simulink model "System_TC6"  (R2015b)
settings: Solver=FixedStepAuto  StartTime=0.0  StopTime=20  FixedStep=0.1  RelTol=1e-3
model workspace: external: MAT-File System_TC6.mat (data not in the file)
libraries: libTLAsserts x16, libAsserts x10
settings Model: Creator=Deepak  LastModifiedBy=Deepak

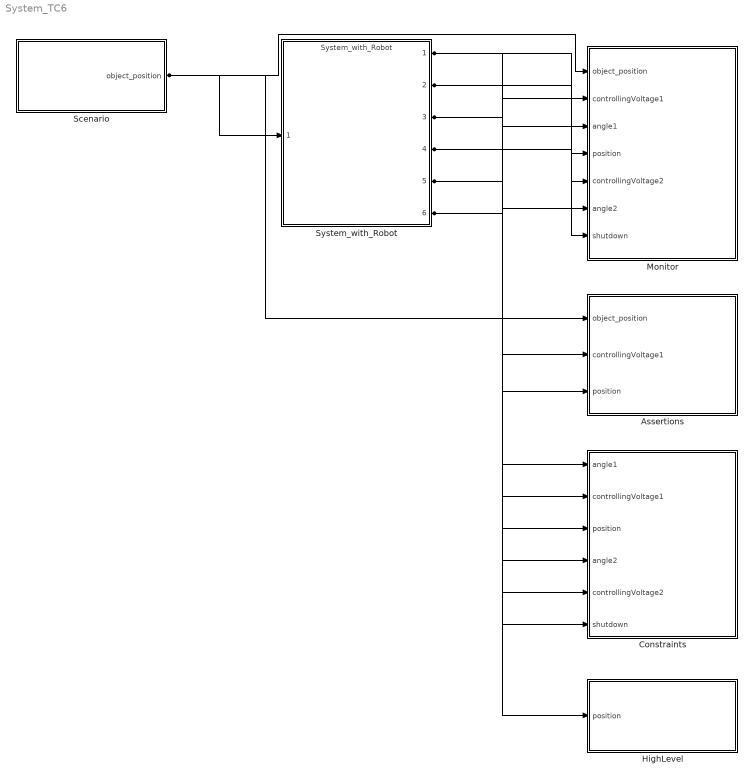
== system System_TC6 ==
  Assertions : Subsystem
  Constraints : Subsystem
  HighLevel : Subsystem
  Monitor : Subsystem
  Scenario : Subsystem
  System_with_Robot : ModelReference  ModelNameDialog=System_with_Robot  SimulationMode=Normal  ModelReferenceVersion=1.26  CopyOfModelName=System_with_Robot
  wires:
  Scenario/1(object_position) -> System_with_Robot/1, Monitor/1(object_position), Assertions/1(object_position)
  System_with_Robot/3 -> Monitor/2(controllingVoltage1), Assertions/2(controllingVoltage1), Constraints/2(controllingVoltage1)
  System_with_Robot/5 -> Monitor/3(angle1), Constraints/1(angle1)
  System_with_Robot/1 -> Monitor/4(position), Assertions/3(position), Constraints/3(position), HighLevel/1(position)
  System_with_Robot/4 -> Monitor/5(controllingVoltage2), Constraints/5(controllingVoltage2)
  System_with_Robot/6 -> Monitor/6(angle2), Constraints/4(angle2)
  System_with_Robot/2 -> Monitor/7(shutdown), Constraints/6(shutdown)

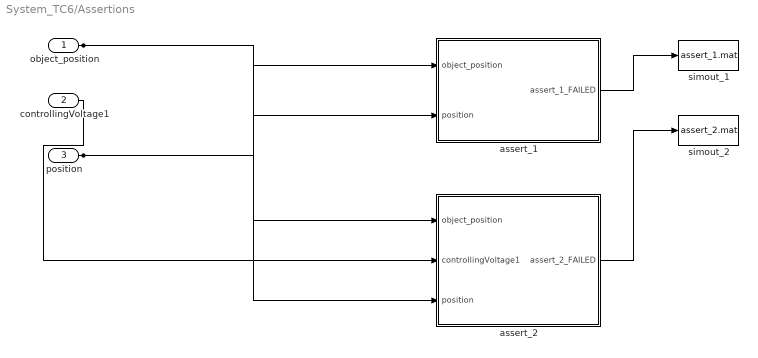
== system System_TC6/Assertions ==
  object_position : Inport
  controllingVoltage1 : Inport  Port=2
  position : Inport  Port=3
  assert_1 : Subsystem
  assert_2 : Subsystem
  simout_1 : ToFile  Filename=assert_1.mat  MatrixName=assert_1  SaveFormat=Timeseries
  simout_2 : ToFile  Filename=assert_2.mat  MatrixName=assert_2  SaveFormat=Timeseries
  wires:
  object_position/1 -> assert_1/1(object_position), assert_2/1(object_position)
  position/1 -> assert_1/2(position), assert_2/3(position)
  assert_1/1(assert_1_FAILED) -> simout_1/1
  controllingVoltage1/1 -> assert_2/2(controllingVoltage1)
  assert_2/1(assert_2_FAILED) -> simout_2/1

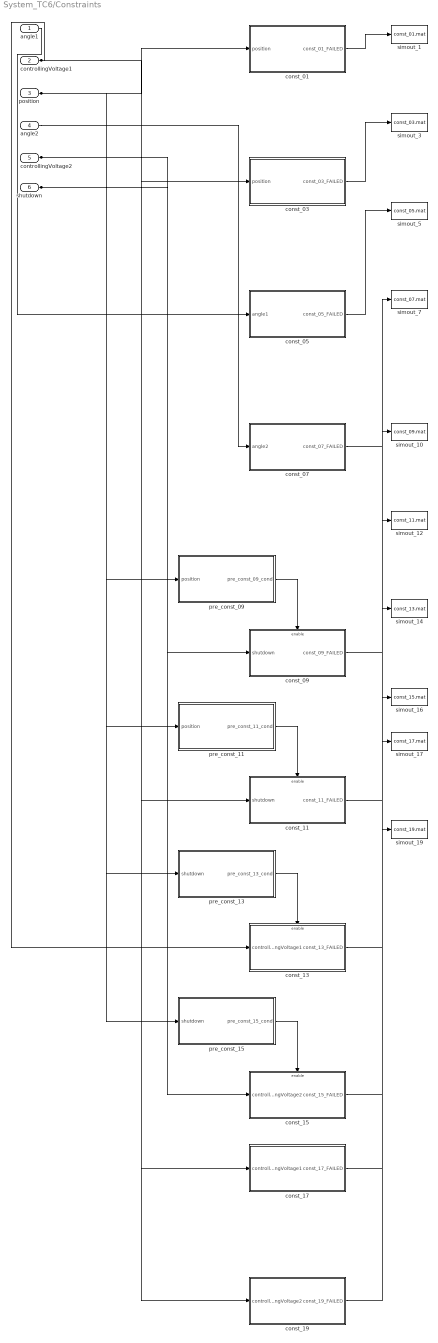
== system System_TC6/Constraints ==
  angle1 : Inport
  controllingVoltage1 : Inport  Port=2
  position : Inport  Port=3
  angle2 : Inport  Port=4
  controllingVoltage2 : Inport  Port=5
  shutdown : Inport  Port=6
  const_01 : Subsystem
  const_03 : Subsystem
  const_05 : Subsystem
  const_07 : Subsystem
  const_09 : Subsystem
  const_11 : Subsystem
  const_13 : Subsystem
  const_15 : Subsystem
  const_17 : Subsystem
  const_19 : Subsystem
  pre_const_09 : Subsystem
  pre_const_11 : Subsystem
  pre_const_13 : Subsystem
  pre_const_15 : Subsystem
  simout_1 : ToFile  Filename=const_01.mat  MatrixName=const_01  SaveFormat=Timeseries
  simout_10 : ToFile  Filename=const_09.mat  MatrixName=const_09  SaveFormat=Timeseries
  simout_12 : ToFile  Filename=const_11.mat  MatrixName=const_11  SaveFormat=Timeseries
  simout_14 : ToFile  Filename=const_13.mat  MatrixName=const_13  SaveFormat=Timeseries
  simout_16 : ToFile  Filename=const_15.mat  MatrixName=const_15  SaveFormat=Timeseries
  simout_17 : ToFile  Filename=const_17.mat  MatrixName=const_17  SaveFormat=Timeseries
  simout_19 : ToFile  Filename=const_19.mat  MatrixName=const_19  SaveFormat=Timeseries
  simout_3 : ToFile  Filename=const_03.mat  MatrixName=const_03  SaveFormat=Timeseries
  simout_5 : ToFile  Filename=const_05.mat  MatrixName=const_05  SaveFormat=Timeseries
  simout_7 : ToFile  Filename=const_07.mat  MatrixName=const_07  SaveFormat=Timeseries
  wires:
  position/1 -> const_01/1(position), const_03/1(position), pre_const_09/1(position), pre_const_11/1(position)
  const_01/1(const_01_FAILED) -> simout_1/1
  const_03/1(const_03_FAILED) -> simout_3/1
  angle1/1 -> const_05/1(angle1)
  const_05/1(const_05_FAILED) -> simout_5/1
  angle2/1 -> const_07/1(angle2)
  const_07/1(const_07_FAILED) -> simout_7/1
  pre_const_09/1(pre_const_09_cond) -> const_09/Enable
  shutdown/1 -> const_09/1(shutdown), const_11/1(shutdown), pre_const_13/1(shutdown), pre_const_15/1(shutdown)
  const_09/1(const_09_FAILED) -> simout_10/1
  pre_const_11/1(pre_const_11_cond) -> const_11/Enable
  const_11/1(const_11_FAILED) -> simout_12/1
  pre_const_13/1(pre_const_13_cond) -> const_13/Enable
  controllingVoltage1/1 -> const_13/1(controllingVoltage1), const_17/1(controllingVoltage1)
  const_13/1(const_13_FAILED) -> simout_14/1
  pre_const_15/1(pre_const_15_cond) -> const_15/Enable
  controllingVoltage2/1 -> const_15/1(controllingVoltage2), const_19/1(controllingVoltage2)
  const_15/1(const_15_FAILED) -> simout_16/1
  const_17/1(const_17_FAILED) -> simout_17/1
  const_19/1(const_19_FAILED) -> simout_19/1

== system System_TC6/HighLevel ==
  position : Inport
  highlevel_1 : Subsystem
  simout_1 : ToFile  Filename=highlevel_1.mat  MatrixName=highlevel_1  SaveFormat=Timeseries
  wires:
  position/1 -> highlevel_1/1(position)
  highlevel_1/1(highlevel_1_FAILED) -> simout_1/1

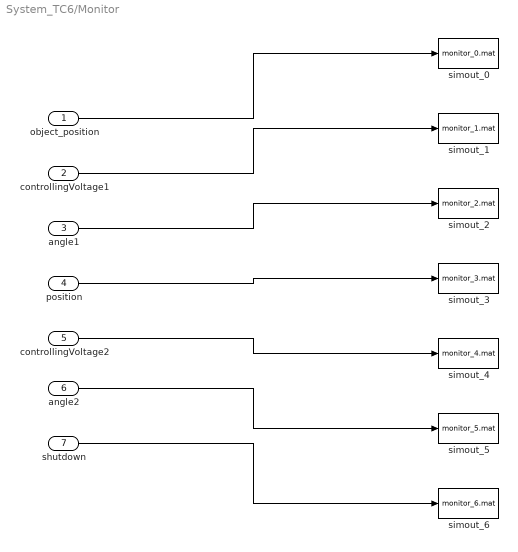
== system System_TC6/Monitor ==
  object_position : Inport
  controllingVoltage1 : Inport  Port=2
  angle1 : Inport  Port=3
  position : Inport  Port=4
  controllingVoltage2 : Inport  Port=5
  angle2 : Inport  Port=6
  shutdown : Inport  Port=7
  simout_0 : ToFile  Filename=monitor_0.mat  MatrixName=object_position  SaveFormat=Timeseries
  simout_1 : ToFile  Filename=monitor_1.mat  MatrixName=controllingVoltage1  SaveFormat=Timeseries
  simout_2 : ToFile  Filename=monitor_2.mat  MatrixName=angle1  SaveFormat=Timeseries
  simout_3 : ToFile  Filename=monitor_3.mat  MatrixName=position  SaveFormat=Timeseries
  simout_4 : ToFile  Filename=monitor_4.mat  MatrixName=controllingVoltage2  SaveFormat=Timeseries
  simout_5 : ToFile  Filename=monitor_5.mat  MatrixName=angle2  SaveFormat=Timeseries
  simout_6 : ToFile  Filename=monitor_6.mat  MatrixName=shutdown  SaveFormat=Timeseries
  wires:
  object_position/1 -> simout_0/1
  controllingVoltage1/1 -> simout_1/1
  angle1/1 -> simout_2/1
  position/1 -> simout_3/1
  controllingVoltage2/1 -> simout_4/1
  angle2/1 -> simout_5/1
  shutdown/1 -> simout_6/1

== system System_TC6/Scenario ==
  Scenario : Stateflow chart  TreatAsAtomicUnit=on
  clock : Clock
  object_position : Outport
  wires:
  Scenario/1(object_position) -> object_position/1
  clock/1 -> Scenario/1(clk)

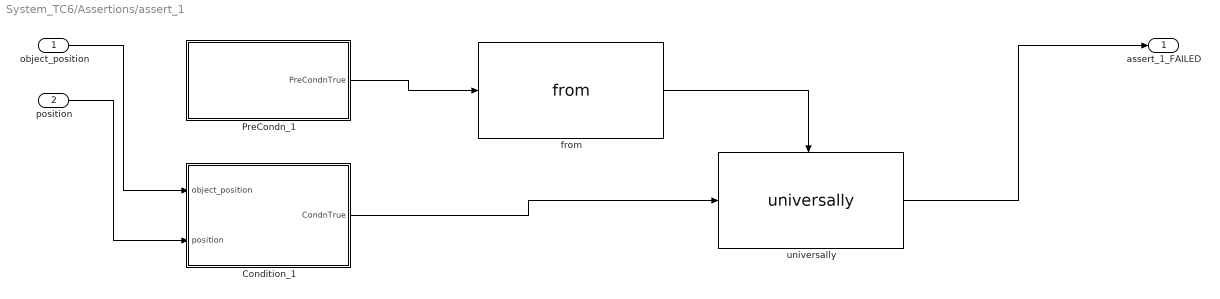
== system System_TC6/Assertions/assert_1 ==
  object_position : Inport
  position : Inport  Port=2
  Condition_1 : Subsystem
  PreCondn_1 : Subsystem
  from : libTLAsserts/from
  universally : libTLAsserts/universally
  assert_1_FAILED : Outport
  wires:
  object_position/1 -> Condition_1/1(object_position)
  position/1 -> Condition_1/2(position)
  PreCondn_1/1(PreCondnTrue) -> from/1
  Condition_1/1(CondnTrue) -> universally/1
  from/1 -> universally/Enable
  universally/1 -> assert_1_FAILED/1

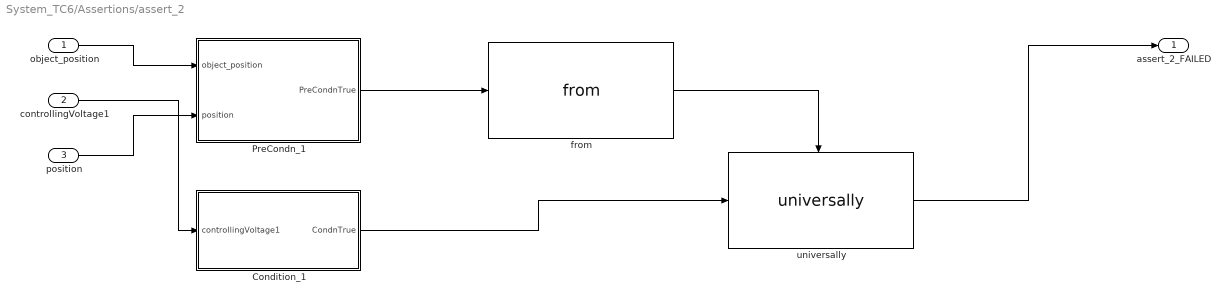
== system System_TC6/Assertions/assert_2 ==
  object_position : Inport
  controllingVoltage1 : Inport  Port=2
  position : Inport  Port=3
  Condition_1 : Subsystem
  PreCondn_1 : Subsystem
  from : libTLAsserts/from
  universally : libTLAsserts/universally
  assert_2_FAILED : Outport
  wires:
  object_position/1 -> PreCondn_1/1(object_position)
  position/1 -> PreCondn_1/2(position)
  controllingVoltage1/1 -> Condition_1/1(controllingVoltage1)
  PreCondn_1/1(PreCondnTrue) -> from/1
  Condition_1/1(CondnTrue) -> universally/1
  from/1 -> universally/Enable
  universally/1 -> assert_2_FAILED/1

== system System_TC6/Constraints/const_01 ==
  position : Inport
  Condition_1 : Subsystem
  globally : libTLAsserts/globally
  universally : libTLAsserts/universally
  const_01_FAILED : Outport
  wires:
  position/1 -> Condition_1/1(position)
  Condition_1/1(CondnTrue) -> universally/1
  globally/1 -> universally/Enable
  universally/1 -> const_01_FAILED/1

== system System_TC6/Constraints/const_03 ==
  position : Inport
  Condition_1 : Subsystem
  globally : libTLAsserts/globally
  universally : libTLAsserts/universally
  const_03_FAILED : Outport
  wires:
  position/1 -> Condition_1/1(position)
  Condition_1/1(CondnTrue) -> universally/1
  globally/1 -> universally/Enable
  universally/1 -> const_03_FAILED/1

== system System_TC6/Constraints/const_05 ==
  angle1 : Inport
  Condition_1 : Subsystem
  globally : libTLAsserts/globally
  universally : libTLAsserts/universally
  const_05_FAILED : Outport
  wires:
  angle1/1 -> Condition_1/1(angle1)
  Condition_1/1(CondnTrue) -> universally/1
  globally/1 -> universally/Enable
  universally/1 -> const_05_FAILED/1

== system System_TC6/Constraints/const_07 ==
  angle2 : Inport
  Condition_1 : Subsystem
  globally : libTLAsserts/globally
  universally : libTLAsserts/universally
  const_07_FAILED : Outport
  wires:
  angle2/1 -> Condition_1/1(angle2)
  Condition_1/1(CondnTrue) -> universally/1
  globally/1 -> universally/Enable
  universally/1 -> const_07_FAILED/1

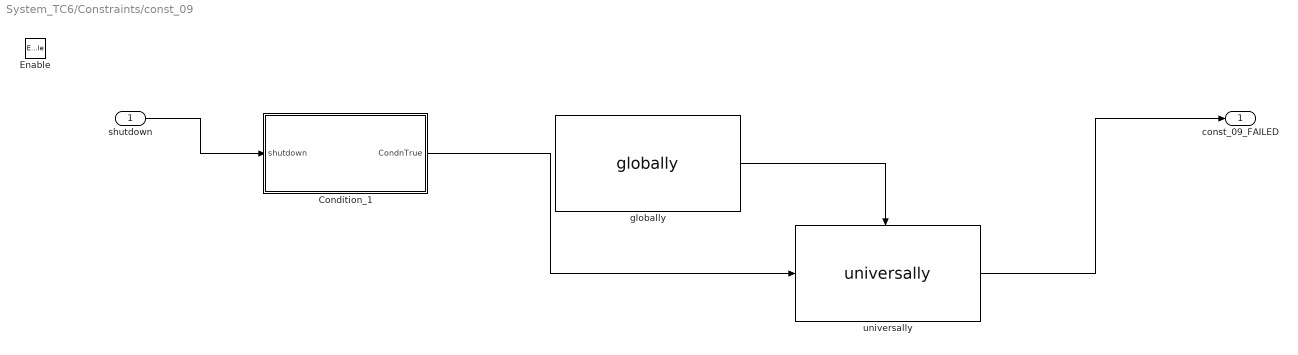
== system System_TC6/Constraints/const_09 ==
  shutdown : Inport
  Enable : EnablePort
  Condition_1 : Subsystem
  globally : libAsserts/globally
  universally : libAsserts/universally
  const_09_FAILED : Outport
  wires:
  shutdown/1 -> Condition_1/1(shutdown)
  Condition_1/1(CondnTrue) -> universally/1
  universally/1 -> const_09_FAILED/1
  globally/1 -> universally/Enable

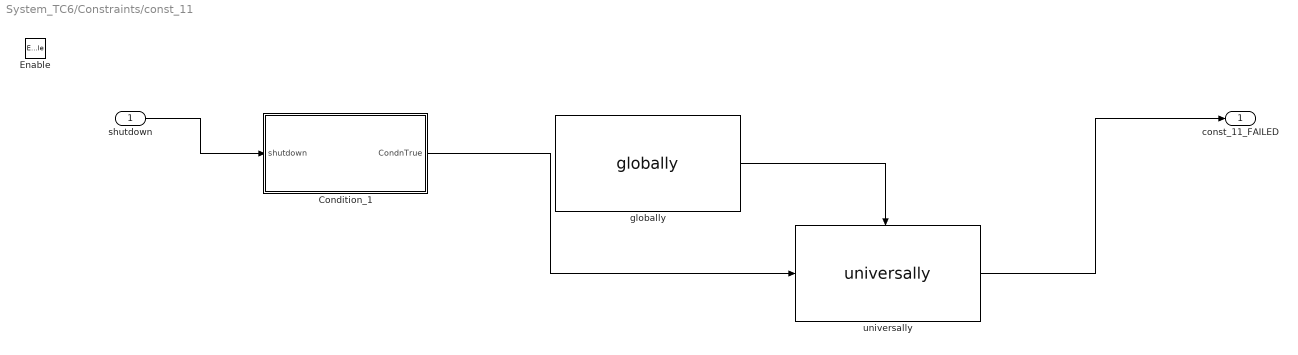
== system System_TC6/Constraints/const_11 ==
  shutdown : Inport
  Enable : EnablePort
  Condition_1 : Subsystem
  globally : libAsserts/globally
  universally : libAsserts/universally
  const_11_FAILED : Outport
  wires:
  shutdown/1 -> Condition_1/1(shutdown)
  Condition_1/1(CondnTrue) -> universally/1
  universally/1 -> const_11_FAILED/1
  globally/1 -> universally/Enable

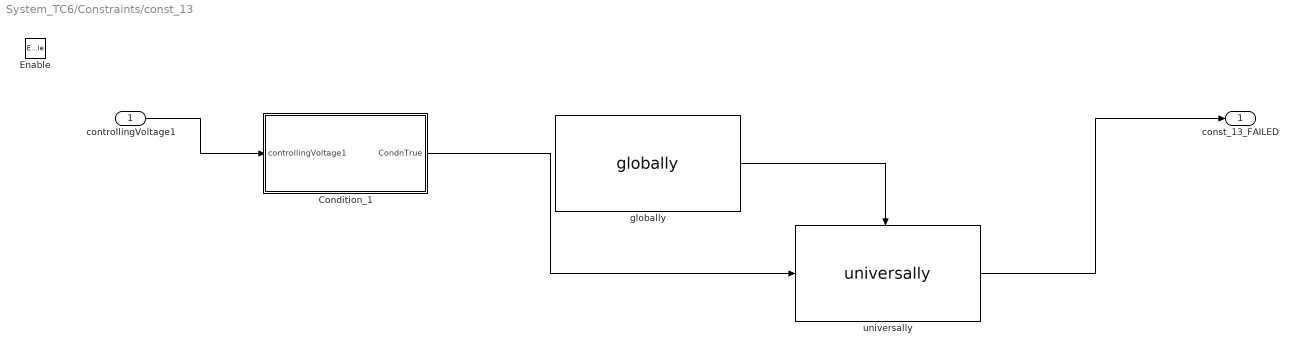
== system System_TC6/Constraints/const_13 ==
  controllingVoltage1 : Inport
  Enable : EnablePort
  Condition_1 : Subsystem
  globally : libAsserts/globally
  universally : libAsserts/universally
  const_13_FAILED : Outport
  wires:
  controllingVoltage1/1 -> Condition_1/1(controllingVoltage1)
  Condition_1/1(CondnTrue) -> universally/1
  universally/1 -> const_13_FAILED/1
  globally/1 -> universally/Enable

== system System_TC6/Constraints/const_15 ==
  controllingVoltage2 : Inport
  Enable : EnablePort
  Condition_1 : Subsystem
  globally : libAsserts/globally
  universally : libAsserts/universally
  const_15_FAILED : Outport
  wires:
  controllingVoltage2/1 -> Condition_1/1(controllingVoltage2)
  Condition_1/1(CondnTrue) -> universally/1
  universally/1 -> const_15_FAILED/1
  globally/1 -> universally/Enable

== system System_TC6/Constraints/const_17 ==
  controllingVoltage1 : Inport
  Condition_1 : Subsystem
  globally : libTLAsserts/globally
  universally : libTLAsserts/universally
  const_17_FAILED : Outport
  wires:
  controllingVoltage1/1 -> Condition_1/1(controllingVoltage1)
  Condition_1/1(CondnTrue) -> universally/1
  globally/1 -> universally/Enable
  universally/1 -> const_17_FAILED/1

== system System_TC6/Constraints/const_19 ==
  controllingVoltage2 : Inport
  Condition_1 : Subsystem
  globally : libTLAsserts/globally
  universally : libTLAsserts/universally
  const_19_FAILED : Outport
  wires:
  controllingVoltage2/1 -> Condition_1/1(controllingVoltage2)
  Condition_1/1(CondnTrue) -> universally/1
  globally/1 -> universally/Enable
  universally/1 -> const_19_FAILED/1

== system System_TC6/Constraints/pre_const_09 ==
  position : Inport
  GreaterExpression_3.0_1.0 : RelationalOperator  Operator=>  OutDataTypeStr=boolean
  NumberLiteral_1.0_1.0 : Constant
  NumberLiteral_1.0_2.0 : Constant  Value=6
  PortItemRefTarget_1.0_1.0 : MultiPortSwitch  Inputs=1
  pre_const_09_cond : Outport
  wires:
  NumberLiteral_1.0_1.0/1 -> PortItemRefTarget_1.0_1.0/1
  position/1 -> PortItemRefTarget_1.0_1.0/2
  PortItemRefTarget_1.0_1.0/1 -> GreaterExpression_3.0_1.0/1
  NumberLiteral_1.0_2.0/1 -> GreaterExpression_3.0_1.0/2
  GreaterExpression_3.0_1.0/1 -> pre_const_09_cond/1

== system System_TC6/Constraints/pre_const_11 ==
  position : Inport
  GreaterExpression_3.0_1.0 : RelationalOperator  Operator=>  OutDataTypeStr=boolean
  NumberLiteral_1.0_1.0 : Constant  Value=2
  NumberLiteral_1.0_2.0 : Constant  Value=6
  PortItemRefTarget_1.0_1.0 : MultiPortSwitch  Inputs=1
  pre_const_11_cond : Outport
  wires:
  NumberLiteral_1.0_1.0/1 -> PortItemRefTarget_1.0_1.0/1
  position/1 -> PortItemRefTarget_1.0_1.0/2
  PortItemRefTarget_1.0_1.0/1 -> GreaterExpression_3.0_1.0/1
  NumberLiteral_1.0_2.0/1 -> GreaterExpression_3.0_1.0/2
  GreaterExpression_3.0_1.0/1 -> pre_const_11_cond/1

== system System_TC6/Constraints/pre_const_13 ==
  shutdown : Inport
  pre_const_13_cond : Outport
  wires:
  shutdown/1 -> pre_const_13_cond/1

== system System_TC6/Constraints/pre_const_15 ==
  shutdown : Inport
  pre_const_15_cond : Outport
  wires:
  shutdown/1 -> pre_const_15_cond/1

== system System_TC6/HighLevel/highlevel_1 ==
  position : Inport
  Condition_1 : Subsystem
  globally : libAsserts/globally
  universally : libAsserts/universally
  highlevel_1_FAILED : Outport
  wires:
  position/1 -> Condition_1/1(position)
  Condition_1/1(CondnTrue) -> universally/1
  universally/1 -> highlevel_1_FAILED/1
  globally/1 -> universally/Enable

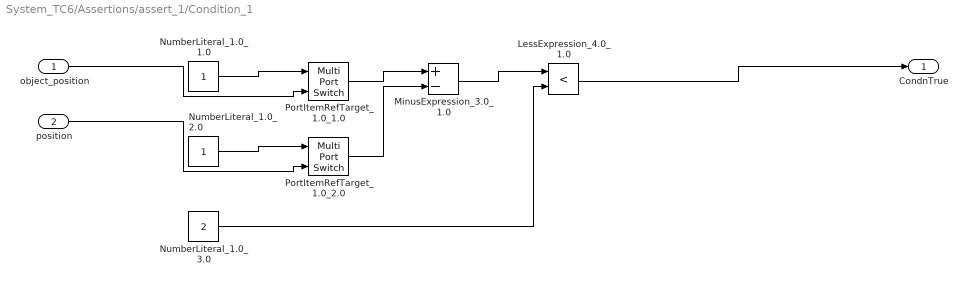
== system System_TC6/Assertions/assert_1/Condition_1 ==
  object_position : Inport
  position : Inport  Port=2
  LessExpression_4.0_1.0 : RelationalOperator  Operator=<  OutDataTypeStr=boolean
  MinusExpression_3.0_1.0 : Sum  Inputs=+-
  NumberLiteral_1.0_1.0 : Constant
  NumberLiteral_1.0_2.0 : Constant
  NumberLiteral_1.0_3.0 : Constant  Value=2
  PortItemRefTarget_1.0_1.0 : MultiPortSwitch  Inputs=1
  PortItemRefTarget_1.0_2.0 : MultiPortSwitch  Inputs=1
  CondnTrue : Outport
  wires:
  NumberLiteral_1.0_1.0/1 -> PortItemRefTarget_1.0_1.0/1
  object_position/1 -> PortItemRefTarget_1.0_1.0/2
  NumberLiteral_1.0_2.0/1 -> PortItemRefTarget_1.0_2.0/1
  position/1 -> PortItemRefTarget_1.0_2.0/2
  PortItemRefTarget_1.0_1.0/1 -> MinusExpression_3.0_1.0/1
  PortItemRefTarget_1.0_2.0/1 -> MinusExpression_3.0_1.0/2
  MinusExpression_3.0_1.0/1 -> LessExpression_4.0_1.0/1
  NumberLiteral_1.0_3.0/1 -> LessExpression_4.0_1.0/2
  LessExpression_4.0_1.0/1 -> CondnTrue/1

== system System_TC6/Assertions/assert_1/PreCondn_1 ==
  AnnotatedExpression_2.0_1.0 : RelationalOperator  OutDataTypeStr=boolean
  NumberLiteral_1.0_1.0 : Constant  Value=5
  clock : Clock
  PreCondnTrue : Outport
  wires:
  clock/1 -> AnnotatedExpression_2.0_1.0/1
  NumberLiteral_1.0_1.0/1 -> AnnotatedExpression_2.0_1.0/2
  AnnotatedExpression_2.0_1.0/1 -> PreCondnTrue/1

== system System_TC6/Assertions/assert_2/Condition_1 ==
  controllingVoltage1 : Inport
  LessExpression_2.0_1.0 : RelationalOperator  Operator=<  OutDataTypeStr=boolean
  NumberLiteral_1.0_1.0 : Constant  Value=2
  CondnTrue : Outport
  wires:
  controllingVoltage1/1 -> LessExpression_2.0_1.0/1
  NumberLiteral_1.0_1.0/1 -> LessExpression_2.0_1.0/2
  LessExpression_2.0_1.0/1 -> CondnTrue/1

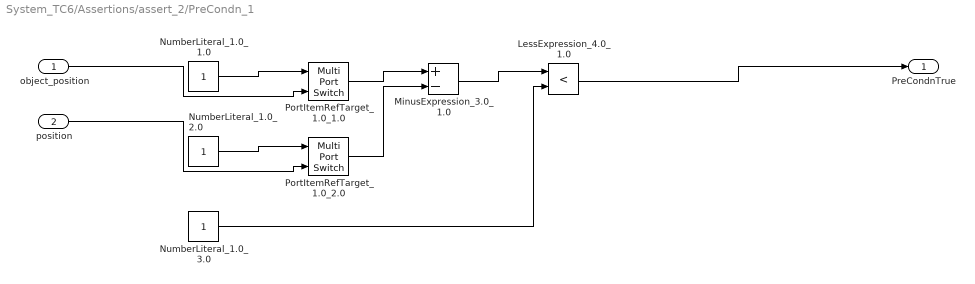
== system System_TC6/Assertions/assert_2/PreCondn_1 ==
  object_position : Inport
  position : Inport  Port=2
  LessExpression_4.0_1.0 : RelationalOperator  Operator=<  OutDataTypeStr=boolean
  MinusExpression_3.0_1.0 : Sum  Inputs=+-
  NumberLiteral_1.0_1.0 : Constant
  NumberLiteral_1.0_2.0 : Constant
  NumberLiteral_1.0_3.0 : Constant
  PortItemRefTarget_1.0_1.0 : MultiPortSwitch  Inputs=1
  PortItemRefTarget_1.0_2.0 : MultiPortSwitch  Inputs=1
  PreCondnTrue : Outport
  wires:
  NumberLiteral_1.0_1.0/1 -> PortItemRefTarget_1.0_1.0/1
  object_position/1 -> PortItemRefTarget_1.0_1.0/2
  NumberLiteral_1.0_2.0/1 -> PortItemRefTarget_1.0_2.0/1
  position/1 -> PortItemRefTarget_1.0_2.0/2
  PortItemRefTarget_1.0_1.0/1 -> MinusExpression_3.0_1.0/1
  PortItemRefTarget_1.0_2.0/1 -> MinusExpression_3.0_1.0/2
  MinusExpression_3.0_1.0/1 -> LessExpression_4.0_1.0/1
  NumberLiteral_1.0_3.0/1 -> LessExpression_4.0_1.0/2
  LessExpression_4.0_1.0/1 -> PreCondnTrue/1

== system System_TC6/Constraints/const_01/Condition_1 ==
  position : Inport
  LessEqualsExpression_3.0_1.0 : RelationalOperator  Operator=<=  OutDataTypeStr=boolean
  NumberLiteral_1.0_1.0 : Constant
  NumberLiteral_1.0_2.0 : Constant  Value=6
  PortItemRefTarget_1.0_1.0 : MultiPortSwitch  Inputs=1
  CondnTrue : Outport
  wires:
  NumberLiteral_1.0_1.0/1 -> PortItemRefTarget_1.0_1.0/1
  position/1 -> PortItemRefTarget_1.0_1.0/2
  PortItemRefTarget_1.0_1.0/1 -> LessEqualsExpression_3.0_1.0/1
  NumberLiteral_1.0_2.0/1 -> LessEqualsExpression_3.0_1.0/2
  LessEqualsExpression_3.0_1.0/1 -> CondnTrue/1

== system System_TC6/Constraints/const_03/Condition_1 ==
  position : Inport
  LessEqualsExpression_3.0_1.0 : RelationalOperator  Operator=<=  OutDataTypeStr=boolean
  NumberLiteral_1.0_1.0 : Constant  Value=2
  NumberLiteral_1.0_2.0 : Constant  Value=6
  PortItemRefTarget_1.0_1.0 : MultiPortSwitch  Inputs=1
  CondnTrue : Outport
  wires:
  NumberLiteral_1.0_1.0/1 -> PortItemRefTarget_1.0_1.0/1
  position/1 -> PortItemRefTarget_1.0_1.0/2
  PortItemRefTarget_1.0_1.0/1 -> LessEqualsExpression_3.0_1.0/1
  NumberLiteral_1.0_2.0/1 -> LessEqualsExpression_3.0_1.0/2
  LessEqualsExpression_3.0_1.0/1 -> CondnTrue/1

== system System_TC6/Constraints/const_05/Condition_1 ==
  angle1 : Inport
  LessEqualsExpression_2.0_1.0 : RelationalOperator  Operator=<=  OutDataTypeStr=boolean
  NumberLiteral_1.0_1.0 : Constant  Value=135
  CondnTrue : Outport
  wires:
  angle1/1 -> LessEqualsExpression_2.0_1.0/1
  NumberLiteral_1.0_1.0/1 -> LessEqualsExpression_2.0_1.0/2
  LessEqualsExpression_2.0_1.0/1 -> CondnTrue/1

== system System_TC6/Constraints/const_07/Condition_1 ==
  angle2 : Inport
  LessEqualsExpression_2.0_1.0 : RelationalOperator  Operator=<=  OutDataTypeStr=boolean
  NumberLiteral_1.0_1.0 : Constant  Value=135
  CondnTrue : Outport
  wires:
  angle2/1 -> LessEqualsExpression_2.0_1.0/1
  NumberLiteral_1.0_1.0/1 -> LessEqualsExpression_2.0_1.0/2
  LessEqualsExpression_2.0_1.0/1 -> CondnTrue/1

== system System_TC6/Constraints/const_09/Condition_1 ==
  shutdown : Inport
  CondnTrue : Outport
  wires:
  shutdown/1 -> CondnTrue/1

== system System_TC6/Constraints/const_11/Condition_1 ==
  shutdown : Inport
  CondnTrue : Outport
  wires:
  shutdown/1 -> CondnTrue/1

== system System_TC6/Constraints/const_13/Condition_1 ==
  controllingVoltage1 : Inport
  EqualsExpression_2.0_1.0 : RelationalOperator  Operator===  OutDataTypeStr=boolean
  NumberLiteral_1.0_1.0 : Constant  Value=0
  CondnTrue : Outport
  wires:
  controllingVoltage1/1 -> EqualsExpression_2.0_1.0/1
  NumberLiteral_1.0_1.0/1 -> EqualsExpression_2.0_1.0/2
  EqualsExpression_2.0_1.0/1 -> CondnTrue/1

== system System_TC6/Constraints/const_15/Condition_1 ==
  controllingVoltage2 : Inport
  EqualsExpression_2.0_1.0 : RelationalOperator  Operator===  OutDataTypeStr=boolean
  NumberLiteral_1.0_1.0 : Constant  Value=0
  CondnTrue : Outport
  wires:
  controllingVoltage2/1 -> EqualsExpression_2.0_1.0/1
  NumberLiteral_1.0_1.0/1 -> EqualsExpression_2.0_1.0/2
  EqualsExpression_2.0_1.0/1 -> CondnTrue/1

== system System_TC6/Constraints/const_17/Condition_1 ==
  controllingVoltage1 : Inport
  LessEqualsExpression_2.0_1.0 : RelationalOperator  Operator=<=  OutDataTypeStr=boolean
  NumberLiteral_1.0_1.0 : Constant  Value=5
  CondnTrue : Outport
  wires:
  controllingVoltage1/1 -> LessEqualsExpression_2.0_1.0/1
  NumberLiteral_1.0_1.0/1 -> LessEqualsExpression_2.0_1.0/2
  LessEqualsExpression_2.0_1.0/1 -> CondnTrue/1

== system System_TC6/Constraints/const_19/Condition_1 ==
  controllingVoltage2 : Inport
  LessEqualsExpression_2.0_1.0 : RelationalOperator  Operator=<=  OutDataTypeStr=boolean
  NumberLiteral_1.0_1.0 : Constant  Value=5
  CondnTrue : Outport
  wires:
  controllingVoltage2/1 -> LessEqualsExpression_2.0_1.0/1
  NumberLiteral_1.0_1.0/1 -> LessEqualsExpression_2.0_1.0/2
  LessEqualsExpression_2.0_1.0/1 -> CondnTrue/1

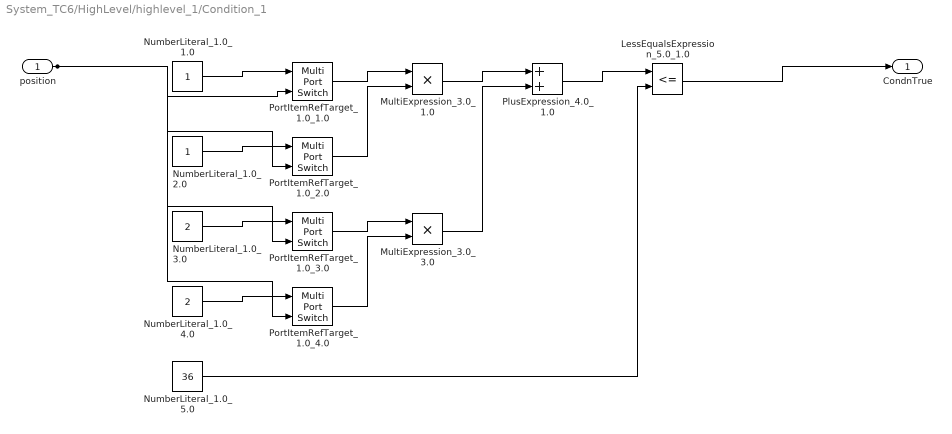
== system System_TC6/HighLevel/highlevel_1/Condition_1 ==
  position : Inport
  LessEqualsExpression_5.0_1.0 : RelationalOperator  Operator=<=  OutDataTypeStr=boolean
  MultiExpression_3.0_1.0 : Product  Inputs=**
  MultiExpression_3.0_3.0 : Product  Inputs=**
  NumberLiteral_1.0_1.0 : Constant
  NumberLiteral_1.0_2.0 : Constant
  NumberLiteral_1.0_3.0 : Constant  Value=2
  NumberLiteral_1.0_4.0 : Constant  Value=2
  NumberLiteral_1.0_5.0 : Constant  Value=36
  PlusExpression_4.0_1.0 : Sum
  PortItemRefTarget_1.0_1.0 : MultiPortSwitch  Inputs=1
  PortItemRefTarget_1.0_2.0 : MultiPortSwitch  Inputs=1
  PortItemRefTarget_1.0_3.0 : MultiPortSwitch  Inputs=1
  PortItemRefTarget_1.0_4.0 : MultiPortSwitch  Inputs=1
  CondnTrue : Outport
  wires:
  NumberLiteral_1.0_1.0/1 -> PortItemRefTarget_1.0_1.0/1
  position/1 -> PortItemRefTarget_1.0_1.0/2, PortItemRefTarget_1.0_2.0/2, PortItemRefTarget_1.0_3.0/2, PortItemRefTarget_1.0_4.0/2
  NumberLiteral_1.0_2.0/1 -> PortItemRefTarget_1.0_2.0/1
  PortItemRefTarget_1.0_1.0/1 -> MultiExpression_3.0_1.0/1
  PortItemRefTarget_1.0_2.0/1 -> MultiExpression_3.0_1.0/2
  NumberLiteral_1.0_3.0/1 -> PortItemRefTarget_1.0_3.0/1
  NumberLiteral_1.0_4.0/1 -> PortItemRefTarget_1.0_4.0/1
  PortItemRefTarget_1.0_3.0/1 -> MultiExpression_3.0_3.0/1
  PortItemRefTarget_1.0_4.0/1 -> MultiExpression_3.0_3.0/2
  MultiExpression_3.0_1.0/1 -> PlusExpression_4.0_1.0/1
  MultiExpression_3.0_3.0/1 -> PlusExpression_4.0_1.0/2
  PlusExpression_4.0_1.0/1 -> LessEqualsExpression_5.0_1.0/1
  NumberLiteral_1.0_5.0/1 -> LessEqualsExpression_5.0_1.0/2
  LessEqualsExpression_5.0_1.0/1 -> CondnTrue/1

== stateflow chart System_TC6/Scenario/Scenario ==
  state Act_System_Step1
    entry: object_position(1) = 5;
    entry: object_position(2) = 5;
  state Act_System_Step2
    entry: object_position(2) = object_position(2) + 0.2;
    entry: Act_System_Step2_stpClk = clk;
  state Act_System_Step3
  (default) -> Act_System_Step1
  Act_System_Step1 -> Act_System_Step2 : [clk > 10]
  Act_System_Step3 -> Act_System_Step2
  Act_System_Step2 -> Act_System_Step3 : [clk - Act_System_Step2_stpClk > 1]
  data: clk input; object_position output =[0;0]; Act_System_Step2_stpClk local
